simulink model "sim12ex5"  (Simulink 2.09)
settings: Solver=ode45  StartTime=0.0  StopTime=25  MaxStep=.1  RelTol=1e-3  AbsTol=1e-3
settings Model: SaveTime=off  SaveOutput=off  ConsistencyChecking=off  RTWTemplateMakefile=grt_vc.tmf

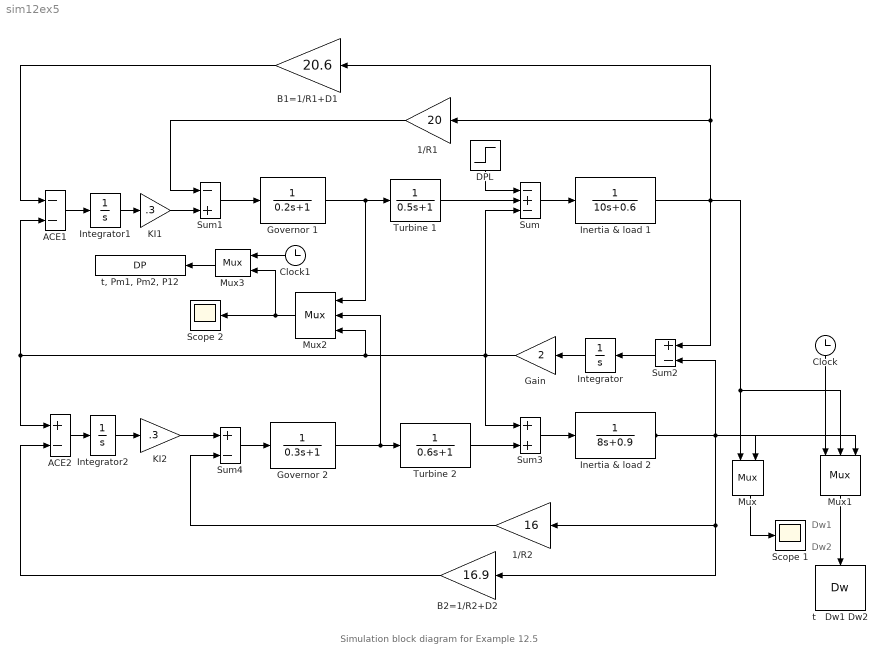
== system sim12ex5 ==
  note: Dw1
  note: Dw2
  note: Simulation block diagram for Example 12.5
  "   Governor 2" : TransferFcn  Numerator=[1]  Denominator="[0.3   1]"
  " Governor 1" : TransferFcn  Numerator=[1]  Denominator="[0.2   1]"
  " Turbine 1" : TransferFcn  Numerator=[1]  Denominator="[0.5  1]"
  1/R1 : Gain  Orientation=left  Gain=20
  "1/R2 " : Gain  Orientation=left  Gain=16
  ACE1 : Sum  Inputs=--
  ACE2 : Sum  Inputs=+-
  B1=1/R1+D1 : Gain  Orientation=left  Gain=20.6
  B2=1/R2+D2 : Gain  Orientation=left  Gain=16.9
  Clock : Clock
      settings: Orientation=down
  Clock1 : Clock
  "DPL " : Step  Orientation=down  Time=100  Before=0.1875  After=.1875
  Gain : Gain  Orientation=left  Gain=2
  "Inertia & load 1 " : TransferFcn  Numerator=[1]  Denominator="[10  0.6]"
  Inertia & load 2 : TransferFcn  Numerator=[1]  Denominator="[8  0.9]"
  Integrator : Integrator  Orientation=left  ExternalReset=none  InitialConditionSource=internal  InitialCondition=0  LimitOutput=off  UpperSaturationLimit=inf  LowerSaturationLimit=-inf  ShowSaturationPort=off  ShowStatePort=off  AbsoluteTolerance=auto
  Integrator1 : Integrator  ExternalReset=none  InitialConditionSource=internal  InitialCondition=0  LimitOutput=off  UpperSaturationLimit=inf  LowerSaturationLimit=-inf  ShowSaturationPort=off  ShowStatePort=off  AbsoluteTolerance=auto
  Integrator2 : Integrator  ExternalReset=none  InitialConditionSource=internal  InitialCondition=0  LimitOutput=off  UpperSaturationLimit=inf  LowerSaturationLimit=-inf  ShowSaturationPort=off  ShowStatePort=off  AbsoluteTolerance=auto
  KI1 : Gain  Gain=.3
  "KI2 " : Gain  Gain=.3
  Mux : Mux  Orientation=down  Inputs=2
  Mux1 : Mux  Orientation=down  Inputs=3
  Mux2 : Mux  Orientation=left  Inputs=3
  Mux3 : Mux  Orientation=left  Inputs=2
  Scope 1 : Scope
      settings: TickLabels=on  TimeRange=auto  YMin=-5  YMax=5  SaveToWorkspace=off  SaveName=ScopeData
  Scope 2 : Scope
      settings: TickLabels=on  TimeRange=auto  YMin=-5  YMax=5  SaveToWorkspace=off  SaveName=ScopeData
  Sum : Sum  Inputs=-+-
  Sum1 : Sum  Inputs=-+
  Sum2 : Sum  Orientation=left  Inputs=+-
  Sum3 : Sum  Inputs=++
  Sum4 : Sum  Inputs=+-
  Turbine 2 : TransferFcn  Numerator=[1]  Denominator="[0.6  1]"
  t   Dw1 Dw2 : ToWorkspace  VariableName=Dw  SampleTime=0
      settings: Orientation=down  Buffer=1000
  "t, Pm1, Pm2, P12" : ToWorkspace  VariableName=DP  SampleTime=0
      settings: Buffer=1000
  wires:
  " Turbine 1"/1 -> Sum/2
  Sum/1 -> "Inertia & load 1 "/1
  Sum1/1 -> " Governor 1"/1
  "DPL "/1 -> Sum/1
  1/R1/1 -> Sum1/1
  Sum2/1 -> Integrator/1
  Integrator/1 -> Gain/1
  Sum3/1 -> Inertia & load 2/1
  Sum4/1 -> "   Governor 2"/1
  Turbine 2/1 -> Sum3/2
  "1/R2 "/1 -> Sum4/2
  Inertia & load 2/1 -> Mux1/3, Mux/2, "1/R2 "/1, B2=1/R2+D2/1, Sum2/2
  Mux1/1 -> t   Dw1 Dw2/1
  Clock/1 -> Mux1/1
  KI1/1 -> Sum1/2
  Integrator1/1 -> KI1/1
  ACE1/1 -> Integrator1/1
  Integrator2/1 -> "KI2 "/1
  ACE2/1 -> Integrator2/1
  "KI2 "/1 -> Sum4/1
  B1=1/R1+D1/1 -> ACE1/1
  B2=1/R2+D2/1 -> ACE2/2
  Mux/1 -> Scope 1/1
  Gain/1 -> Sum/3, Sum3/1, ACE1/2, ACE2/1, Mux2/3
  " Governor 1"/1 -> " Turbine 1"/1, Mux2/1
  "   Governor 2"/1 -> Turbine 2/1, Mux2/2
  "Inertia & load 1 "/1 -> Sum2/1, 1/R1/1, B1=1/R1+D1/1, Mux/1, Mux1/2
  Mux2/1 -> Scope 2/1, Mux3/2
  Clock1/1 -> Mux3/1
  Mux3/1 -> "t, Pm1, Pm2, P12"/1
